simulink model "turbin_img"  (R2012b)
settings: Solver=ode45  StartTime=0.0  StopTime=10.0  RelTol=1e-3
values from neighbouring files (symbols this model uses):
  cp_exh = gamma_exh*cv_exh    (= 980)    [Init_Project1.m]
  dT1 = 1    [Init_Project2.m]
  gamma_exh = 1.4    [Init_Project1.m]
  T_em = mean(T_em)    [Init_Project1.m]
undefined symbols (not defined in the file or in its folder): BSR_max, eta_T_max, TFP_exp, TFP_max
settings Model: Creator=rasme879  LastModifiedBy=rasme879

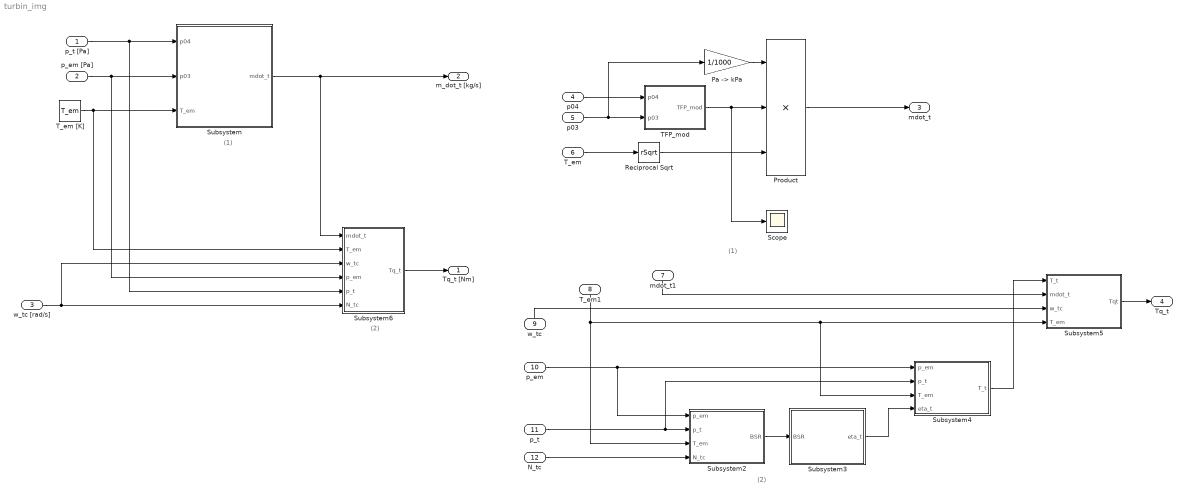
== system turbin_img ==
  note: (2)
  note: (2)
  note: (1)
  note: (1)
  "p_t [Pa] " : Inport
  p_em [Pa] : Inport  Port=2
  w_tc [rad/s] : Inport  Port=3
  p04 : Inport  Port=4
  p03 : Inport  Port=5
  T_em : Inport  Port=6
  mdot_t1 : Inport  Port=7
  T_em1 : Inport  Port=8
  w_tc : Inport  Port=9
  p_em : Inport  Port=10
  p_t : Inport  Port=11
  N_tc : Inport  Port=12
  "Pa -> kPa" : Gain  Gain=1/1000
  Product : Product  Inputs=3
  Reciprocal Sqrt : Sqrt  Operator=rSqrt  SaturateOnIntegerOverflow=on
  Scope : Scope
      settings: YMin=0.001  YMax=0.0055
  Subsystem : Subsystem
  Subsystem2 : Subsystem
  Subsystem3 : Subsystem
  Subsystem4 : Subsystem
  Subsystem5 : Subsystem
  Subsystem6 : Subsystem
  TFP_mod : Subsystem
  T_em [K] : Constant  Value=T_em
  Tq_t [Nm] : Outport
  m_dot_t [kg/s] : Outport  Port=2
  mdot_t : Outport  Port=3
  Tq_t : Outport  Port=4
  wires:
  p_em [Pa]/1 -> Subsystem6/4(p_em), Subsystem/2(p03)
  "p_t [Pa] "/1 -> Subsystem6/5(p_t), Subsystem/1(p04)
  T_em [K]/1 -> Subsystem6/2(T_em), Subsystem/3(T_em)
  Subsystem/1(mdot_t) -> Subsystem6/1(mdot_t), m_dot_t [kg/s]/1
  Subsystem6/1(Tq_t) -> Tq_t [Nm]/1
  w_tc [rad/s]/1 -> Subsystem6/6(N_tc), Subsystem6/3(w_tc)
  Reciprocal Sqrt/1 -> Product/3
  T_em/1 -> Reciprocal Sqrt/1
  TFP_mod/1(TFP_mod) -> Scope/1, Product/2
  p03/1 -> "Pa -> kPa"/1, TFP_mod/2(p03)
  p04/1 -> TFP_mod/1(p04)
  Product/1 -> mdot_t/1
  "Pa -> kPa"/1 -> Product/1
  mdot_t1/1 -> Subsystem5/2(mdot_t)
  w_tc/1 -> Subsystem5/3(w_tc)
  Subsystem5/1(Tqt) -> Tq_t/1
  Subsystem4/1(T_t) -> Subsystem5/1(T_t)
  Subsystem3/1(eta_t) -> Subsystem4/4(eta_t)
  Subsystem2/1(BSR) -> Subsystem3/1(BSR)
  N_tc/1 -> Subsystem2/4(N_tc)
  p_t/1 -> Subsystem4/2(p_t), Subsystem2/2(p_t)
  p_em/1 -> Subsystem2/1(p_em), Subsystem4/1(p_em)
  T_em1/1 -> Subsystem2/3(T_em), Subsystem4/3(T_em), Subsystem5/4(T_em)

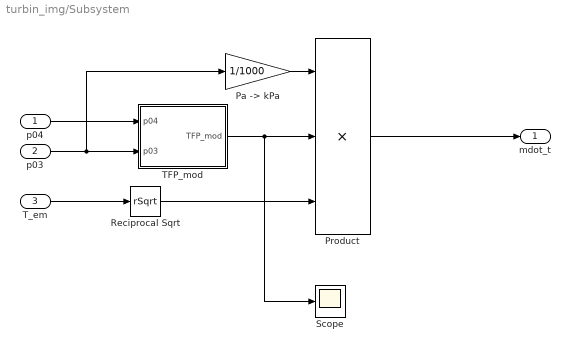
== system turbin_img/Subsystem ==
  p04 : Inport
  p03 : Inport  Port=2
  T_em : Inport  Port=3
  "Pa -> kPa" : Gain  Gain=1/1000
  Product : Product  Inputs=3
  Reciprocal Sqrt : Sqrt  Operator=rSqrt  SaturateOnIntegerOverflow=on
  Scope : Scope
      settings: YMin=0.001  YMax=0.0055  SaveName=ScopeData5
  TFP_mod : Subsystem
  mdot_t : Outport
  wires:
  Reciprocal Sqrt/1 -> Product/3
  T_em/1 -> Reciprocal Sqrt/1
  TFP_mod/1(TFP_mod) -> Scope/1, Product/2
  p03/1 -> "Pa -> kPa"/1, TFP_mod/2(p03)
  p04/1 -> TFP_mod/1(p04)
  Product/1 -> mdot_t/1
  "Pa -> kPa"/1 -> Product/1

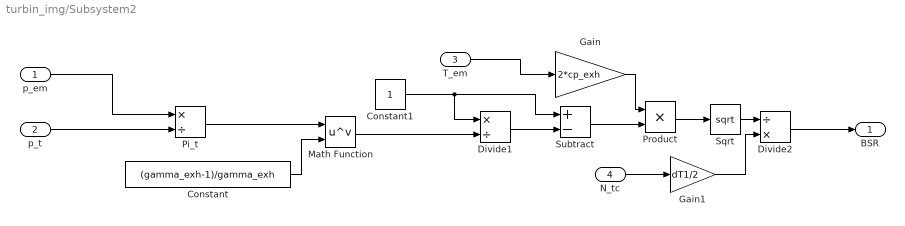
== system turbin_img/Subsystem2 ==
  p_em : Inport
  p_t : Inport  Port=2
  T_em : Inport  Port=3
  N_tc : Inport  Port=4
  Constant : Constant  Value=(gamma_exh-1)/gamma_exh
  Constant1 : Constant
  Divide1 : Product  Inputs=*/
  Divide2 : Product  Inputs=/*
  Gain : Gain  Gain=2*cp_exh
  Gain1 : Gain  Gain=dT1/2
  Math Function : Math  Operator=pow  SaturateOnIntegerOverflow=on
  Pi_t : Product  Inputs=*/
  Product : Product  RndMeth=Zero
  Sqrt : Sqrt  SaturateOnIntegerOverflow=on
  Subtract : Sum  Inputs=+-
  BSR : Outport
  wires:
  Pi_t/1 -> Math Function/1
  Constant/1 -> Math Function/2
  Math Function/1 -> Divide1/2
  Constant1/1 -> Subtract/1, Divide1/1
  Divide1/1 -> Subtract/2
  Product/1 -> Sqrt/1
  Subtract/1 -> Product/2
  Gain/1 -> Product/1
  T_em/1 -> Gain/1
  Sqrt/1 -> Divide2/1
  Divide2/1 -> BSR/1
  Gain1/1 -> Divide2/2
  N_tc/1 -> Gain1/1
  p_t/1 -> Pi_t/2
  p_em/1 -> Pi_t/1

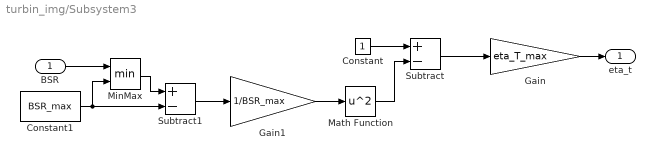
== system turbin_img/Subsystem3 ==
  BSR : Inport
  Constant : Constant
  Constant1 : Constant  Value=BSR_max
  Gain : Gain  Gain=eta_T_max
  Gain1 : Gain  Gain=1/BSR_max
  Math Function : Math  Operator=square  SaturateOnIntegerOverflow=on
  MinMax : MinMax  Inputs=2
  Subtract : Sum  Inputs=+-
  Subtract1 : Sum  Inputs=+-
  eta_t : Outport
  wires:
  Gain/1 -> eta_t/1
  Subtract/1 -> Gain/1
  Constant/1 -> Subtract/1
  Math Function/1 -> Subtract/2
  Gain1/1 -> Math Function/1
  Subtract1/1 -> Gain1/1
  Constant1/1 -> MinMax/2, Subtract1/2
  BSR/1 -> MinMax/1
  MinMax/1 -> Subtract1/1

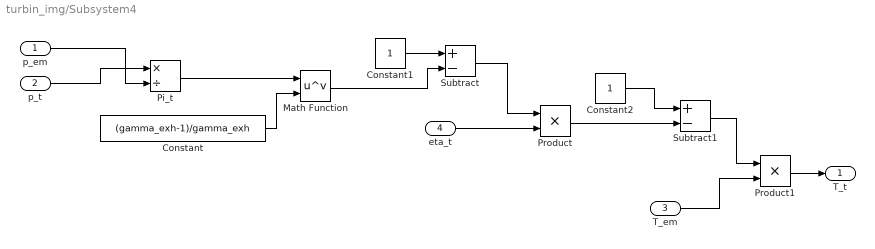
== system turbin_img/Subsystem4 ==
  p_em : Inport
  p_t : Inport  Port=2
  T_em : Inport  Port=3
  eta_t : Inport  Port=4
  Constant : Constant  Value=(gamma_exh-1)/gamma_exh
  Constant1 : Constant
  Constant2 : Constant
  Math Function : Math  Operator=pow  SaturateOnIntegerOverflow=on
  Pi_t : Product  Inputs=*/
  Product : Product  RndMeth=Zero
  Product1 : Product  RndMeth=Zero
  Subtract : Sum  Inputs=+-
  Subtract1 : Sum  Inputs=+-
  T_t : Outport
  wires:
  p_t/1 -> Pi_t/1
  p_em/1 -> Pi_t/2
  Pi_t/1 -> Math Function/1
  Constant/1 -> Math Function/2
  Constant1/1 -> Subtract/1
  Math Function/1 -> Subtract/2
  Subtract/1 -> Product/1
  eta_t/1 -> Product/2
  Constant2/1 -> Subtract1/1
  Product/1 -> Subtract1/2
  Product1/1 -> T_t/1
  Subtract1/1 -> Product1/1
  T_em/1 -> Product1/2

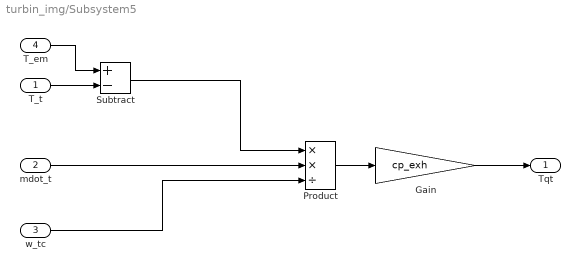
== system turbin_img/Subsystem5 ==
  T_t : Inport
  mdot_t : Inport  Port=2
  w_tc : Inport  Port=3
  T_em : Inport  Port=4
  Gain : Gain  Gain=cp_exh
  Product : Product  Inputs=**/  RndMeth=Zero
  Subtract : Sum  Inputs=+-
  Tqt : Outport
  wires:
  w_tc/1 -> Product/3
  mdot_t/1 -> Product/2
  T_t/1 -> Subtract/2
  T_em/1 -> Subtract/1
  Subtract/1 -> Product/1
  Product/1 -> Gain/1
  Gain/1 -> Tqt/1

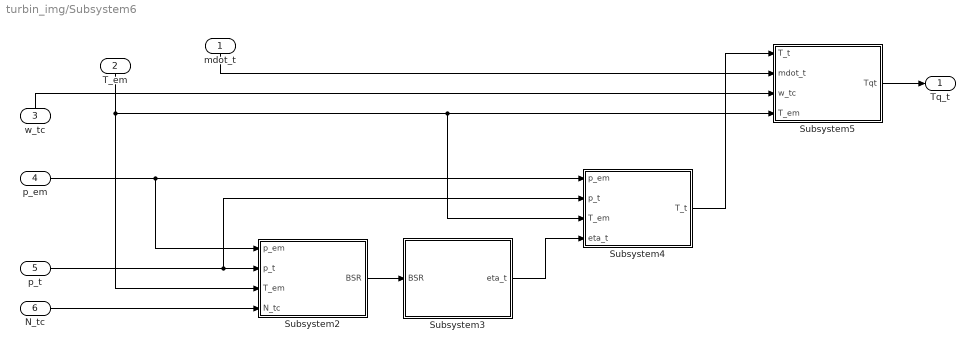
== system turbin_img/Subsystem6 ==
  mdot_t : Inport
  T_em : Inport  Port=2
  w_tc : Inport  Port=3
  p_em : Inport  Port=4
  p_t : Inport  Port=5
  N_tc : Inport  Port=6
  Subsystem2 : Subsystem
  Subsystem3 : Subsystem
  Subsystem4 : Subsystem
  Subsystem5 : Subsystem
  Tq_t : Outport
  wires:
  mdot_t/1 -> Subsystem5/2(mdot_t)
  w_tc/1 -> Subsystem5/3(w_tc)
  Subsystem5/1(Tqt) -> Tq_t/1
  Subsystem4/1(T_t) -> Subsystem5/1(T_t)
  Subsystem3/1(eta_t) -> Subsystem4/4(eta_t)
  Subsystem2/1(BSR) -> Subsystem3/1(BSR)
  N_tc/1 -> Subsystem2/4(N_tc)
  p_t/1 -> Subsystem4/2(p_t), Subsystem2/2(p_t)
  p_em/1 -> Subsystem2/1(p_em), Subsystem4/1(p_em)
  T_em/1 -> Subsystem2/3(T_em), Subsystem4/3(T_em), Subsystem5/4(T_em)

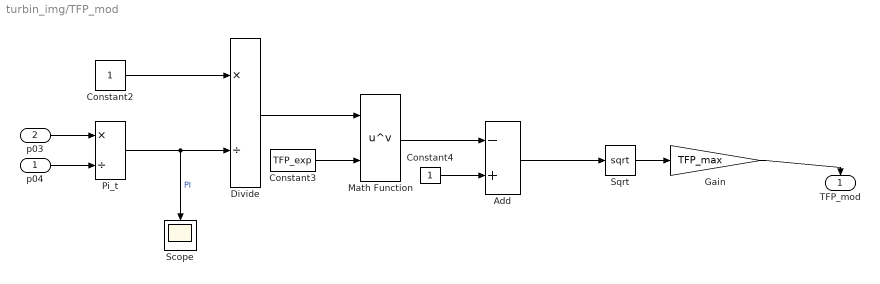
== system turbin_img/TFP_mod ==
  p04 : Inport
  p03 : Inport  Port=2
  Add : Sum  Inputs=-+
  Constant2 : Constant
  Constant3 : Constant  Value=TFP_exp
  Constant4 : Constant
  Divide : Product  Inputs=*/
  Gain : Gain  Gain=TFP_max
  Math Function : Math  Operator=pow  SaturateOnIntegerOverflow=on
  Pi_t : Product  Inputs=*/
  Scope : Scope
      settings: SaveName=ScopeData7
  Sqrt : Sqrt  SaturateOnIntegerOverflow=on
  TFP_mod : Outport
  wires:
  p03/1 -> Pi_t/1
  p04/1 -> Pi_t/2
  Constant2/1 -> Divide/1
  Divide/1 -> Math Function/1
  Constant3/1 -> Math Function/2
  Constant4/1 -> Add/2
  Gain/1 -> TFP_mod/1
  Sqrt/1 -> Gain/1
  Math Function/1 -> Add/1
  Pi_t/1 -> Divide/2, Scope/1  "PI"
  Add/1 -> Sqrt/1

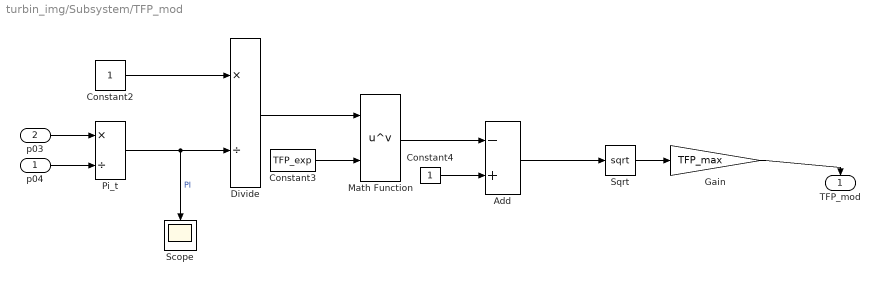
== system turbin_img/Subsystem/TFP_mod ==
  p04 : Inport
  p03 : Inport  Port=2
  Add : Sum  Inputs=-+
  Constant2 : Constant
  Constant3 : Constant  Value=TFP_exp
  Constant4 : Constant
  Divide : Product  Inputs=*/
  Gain : Gain  Gain=TFP_max
  Math Function : Math  Operator=pow  SaturateOnIntegerOverflow=on
  Pi_t : Product  Inputs=*/
  Scope : Scope
      settings: SaveName=ScopeData7
  Sqrt : Sqrt  SaturateOnIntegerOverflow=on
  TFP_mod : Outport
  wires:
  p03/1 -> Pi_t/1
  p04/1 -> Pi_t/2
  Constant2/1 -> Divide/1
  Divide/1 -> Math Function/1
  Constant3/1 -> Math Function/2
  Constant4/1 -> Add/2
  Gain/1 -> TFP_mod/1
  Sqrt/1 -> Gain/1
  Math Function/1 -> Add/1
  Pi_t/1 -> Divide/2, Scope/1  "PI"
  Add/1 -> Sqrt/1

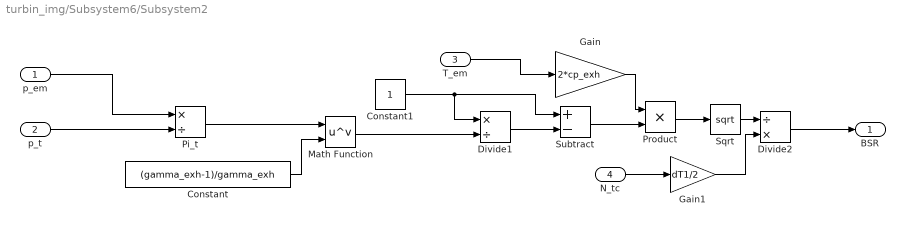
== system turbin_img/Subsystem6/Subsystem2 ==
  p_em : Inport
  p_t : Inport  Port=2
  T_em : Inport  Port=3
  N_tc : Inport  Port=4
  Constant : Constant  Value=(gamma_exh-1)/gamma_exh
  Constant1 : Constant
  Divide1 : Product  Inputs=*/
  Divide2 : Product  Inputs=/*
  Gain : Gain  Gain=2*cp_exh
  Gain1 : Gain  Gain=dT1/2
  Math Function : Math  Operator=pow  SaturateOnIntegerOverflow=on
  Pi_t : Product  Inputs=*/
  Product : Product  RndMeth=Zero
  Sqrt : Sqrt  SaturateOnIntegerOverflow=on
  Subtract : Sum  Inputs=+-
  BSR : Outport
  wires:
  Pi_t/1 -> Math Function/1
  Constant/1 -> Math Function/2
  Math Function/1 -> Divide1/2
  Constant1/1 -> Subtract/1, Divide1/1
  Divide1/1 -> Subtract/2
  Product/1 -> Sqrt/1
  Subtract/1 -> Product/2
  Gain/1 -> Product/1
  T_em/1 -> Gain/1
  Sqrt/1 -> Divide2/1
  Divide2/1 -> BSR/1
  Gain1/1 -> Divide2/2
  N_tc/1 -> Gain1/1
  p_t/1 -> Pi_t/2
  p_em/1 -> Pi_t/1

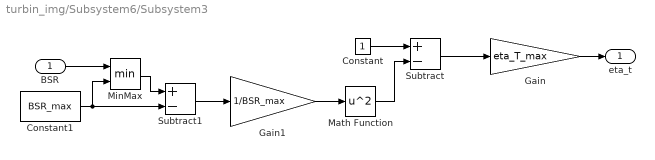
== system turbin_img/Subsystem6/Subsystem3 ==
  BSR : Inport
  Constant : Constant
  Constant1 : Constant  Value=BSR_max
  Gain : Gain  Gain=eta_T_max
  Gain1 : Gain  Gain=1/BSR_max
  Math Function : Math  Operator=square  SaturateOnIntegerOverflow=on
  MinMax : MinMax  Inputs=2
  Subtract : Sum  Inputs=+-
  Subtract1 : Sum  Inputs=+-
  eta_t : Outport
  wires:
  Gain/1 -> eta_t/1
  Subtract/1 -> Gain/1
  Constant/1 -> Subtract/1
  Math Function/1 -> Subtract/2
  Gain1/1 -> Math Function/1
  Subtract1/1 -> Gain1/1
  Constant1/1 -> MinMax/2, Subtract1/2
  BSR/1 -> MinMax/1
  MinMax/1 -> Subtract1/1

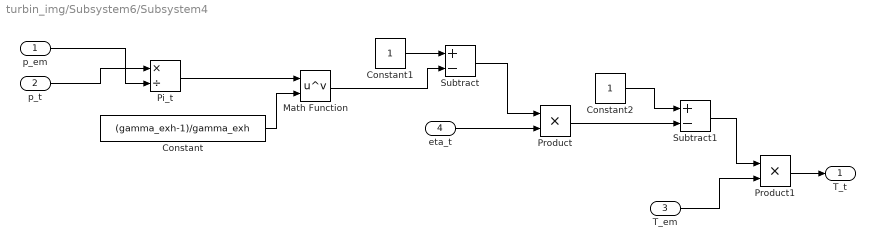
== system turbin_img/Subsystem6/Subsystem4 ==
  p_em : Inport
  p_t : Inport  Port=2
  T_em : Inport  Port=3
  eta_t : Inport  Port=4
  Constant : Constant  Value=(gamma_exh-1)/gamma_exh
  Constant1 : Constant
  Constant2 : Constant
  Math Function : Math  Operator=pow  SaturateOnIntegerOverflow=on
  Pi_t : Product  Inputs=*/
  Product : Product  RndMeth=Zero
  Product1 : Product  RndMeth=Zero
  Subtract : Sum  Inputs=+-
  Subtract1 : Sum  Inputs=+-
  T_t : Outport
  wires:
  p_t/1 -> Pi_t/1
  p_em/1 -> Pi_t/2
  Pi_t/1 -> Math Function/1
  Constant/1 -> Math Function/2
  Constant1/1 -> Subtract/1
  Math Function/1 -> Subtract/2
  Subtract/1 -> Product/1
  eta_t/1 -> Product/2
  Constant2/1 -> Subtract1/1
  Product/1 -> Subtract1/2
  Product1/1 -> T_t/1
  Subtract1/1 -> Product1/1
  T_em/1 -> Product1/2

== system turbin_img/Subsystem6/Subsystem5 ==
  T_t : Inport
  mdot_t : Inport  Port=2
  w_tc : Inport  Port=3
  T_em : Inport  Port=4
  Gain : Gain  Gain=cp_exh
  Product : Product  Inputs=**/  RndMeth=Zero
  Subtract : Sum  Inputs=+-
  Tqt : Outport
  wires:
  w_tc/1 -> Product/3
  mdot_t/1 -> Product/2
  T_t/1 -> Subtract/2
  T_em/1 -> Subtract/1
  Subtract/1 -> Product/1
  Product/1 -> Gain/1
  Gain/1 -> Tqt/1
